simulink model "Model_Based_Design"  (R2024b)
settings: Solver=FixedStepDiscrete  StartTime=0.0  StopTime=0.5  FixedStep=0.1  RelTol=1e-3
libraries: SignalEditorBlockLib x1
settings Model: Creator=USER  LastModifiedBy=USER

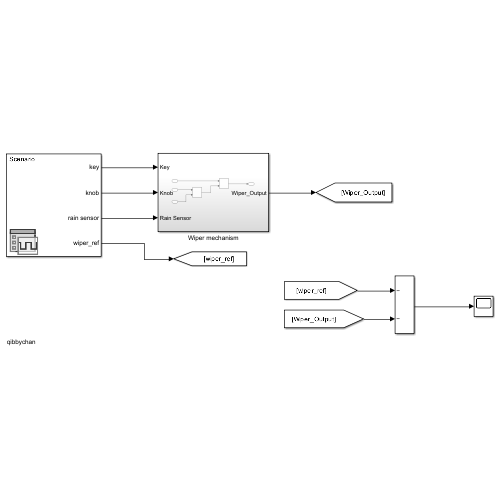
[thumbnail: Simulink's stored preview of the top-level diagram]
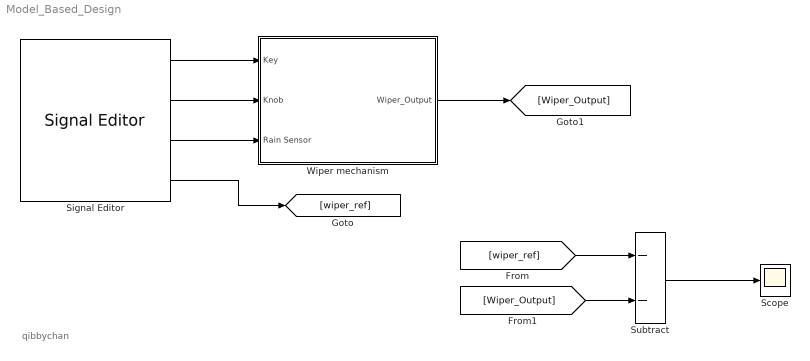
== system Model_Based_Design ==
  note: qibbychan
  Scope : Scope
  Signal Editor : SignalEditorBlockLib/Signal Editor  FileName=car_wiper_mechanism.mat  ActiveScenario=Scenario  ActiveSignal=key  IsBus=off  OutputBusObjectStr=Bus: BusObject  SampleTime=0  Interpolate=off  ZeroCross=off  OutputAfterFinalValue=Setting to zero  Unit=inherit  PreserveSignalName=on  ApplySigPropsToAllScenarios=on  ApplySigPropsToAllSignals=off
  Subtract : Sum  Inputs=--
  Wiper mechanism : Subsystem
  wires:
  Signal Editor/1 -> Wiper mechanism/1(Key)
  Signal Editor/2 -> Wiper mechanism/2(Knob)
  Signal Editor/3 -> Wiper mechanism/3(Rain Sensor)
  Signal Editor/4 -> [wiper_ref]
  Wiper mechanism/1(Wiper_Output) -> [Wiper_Output]
  [wiper_ref] -> Subtract/1
  [Wiper_Output] -> Subtract/2
  Subtract/1 -> Scope/1

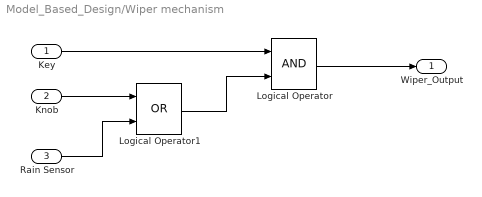
== system Model_Based_Design/Wiper mechanism ==
  Key : Inport
  Knob : Inport  Port=2
  Rain Sensor : Inport  Port=3
  Logical Operator : Logic  AllPortsSameDT=off  OutDataTypeStr=boolean
  Logical Operator1 : Logic  Operator=OR  AllPortsSameDT=off  OutDataTypeStr=boolean
  Wiper_Output : Outport
  wires:
  Logical Operator1/1 -> Logical Operator/2
  Key/1 -> Logical Operator/1
  Logical Operator/1 -> Wiper_Output/1
  Rain Sensor/1 -> Logical Operator1/2
  Knob/1 -> Logical Operator1/1
